simulink model "Aufgabe2_nicht_linear"  (R2025b)
settings: Solver=ode5  StartTime=0.0  StopTime=50  FixedStep=0.05  RelTol=1e-3
settings Model: Creator=henri  LastModifiedBy=henri

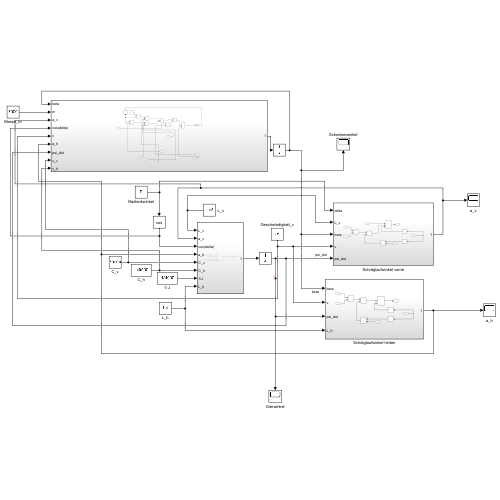
[thumbnail: Simulink's stored preview of the top-level diagram]
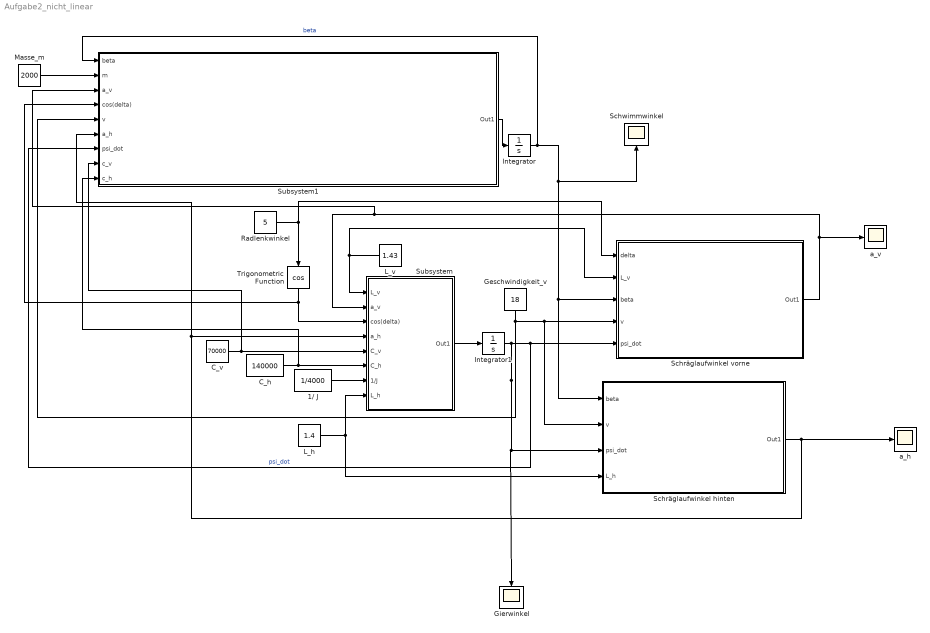
== system Aufgabe2_nicht_linear ==
  1/ J : Constant  Value=1/4000
  C_h : Constant  Value=140000
  C_v : Constant  Value=70000
  Geschwindigkeit_v : Constant  Value=18
  Gierwinkel : Scope
      settings: ActiveDisplayYMinimum=-1.0140786110140794  ActiveDisplayYMaximum=9.1267074991267165
  Integrator : Integrator
  Integrator1 : Integrator
  L_h : Constant  Value=1.4
  L_v : Constant  Value=1.43
  Masse_m : Constant  Value=2000
  Radlenkwinkel : Constant  Value=5
  Schräglaufwinkel hinten : Subsystem
  Schräglaufwinkel vorne : Subsystem
  Schwimmwinkel : Scope
      settings: ActiveDisplayYMinimum=-0.67350842338242578  ActiveDisplayYMaximum=0.35724955186258422
  Subsystem : Subsystem
  Subsystem1 : Subsystem
  Trigonometric Function : Trigonometry  Operator=cos
  a_h : Scope
      settings: ActiveDisplayYMinimum=0.59875782230441044  ActiveDisplayYMaximum=0.7625039748548651  DataLoggingVariableName=ScopeData2
  a_v : Scope
      settings: ActiveDisplayYMinimum=4.248464796495246  ActiveDisplayYMaximum=4.4144687229732016  DataLoggingVariableName=ScopeData3
  wires:
  Trigonometric Function/1 -> Subsystem1/4(cos(delta)), Subsystem/3(cos(delta))
  Radlenkwinkel/1 -> Trigonometric Function/1, Schräglaufwinkel vorne/1(delta)
  L_h/1 -> Subsystem/8(L_h), Schräglaufwinkel hinten/4(L_h)
  Integrator1/1 -> Gierwinkel/1, Schräglaufwinkel hinten/3(psi_dot), Subsystem1/7(psi_dot), Schräglaufwinkel vorne/5(psi_dot)  "psi_dot"
  L_v/1 -> Schräglaufwinkel vorne/2(L_v), Subsystem/1(L_v)
  C_v/1 -> Subsystem1/8(c_v), Subsystem/5(C_v)
  1/ J/1 -> Subsystem/7(1/J)
  Geschwindigkeit_v/1 -> Subsystem1/5(v), Schräglaufwinkel vorne/4(v), Schräglaufwinkel hinten/2(v)
  C_h/1 -> Subsystem1/9(c_h), Subsystem/6(C_h)
  Schräglaufwinkel vorne/1(Out1) -> a_v/1, Subsystem1/3(a_v), Subsystem/2(a_v)
  Subsystem/1(Out1) -> Integrator1/1
  Integrator/1 -> Subsystem1/1(beta), Schwimmwinkel/1, Schräglaufwinkel vorne/3(beta), Schräglaufwinkel hinten/1(beta)  "beta"
  Schräglaufwinkel hinten/1(Out1) -> Subsystem1/6(a_h), Subsystem/4(a_h), a_h/1
  Masse_m/1 -> Subsystem1/2(m)
  Subsystem1/1(Out1) -> Integrator/1

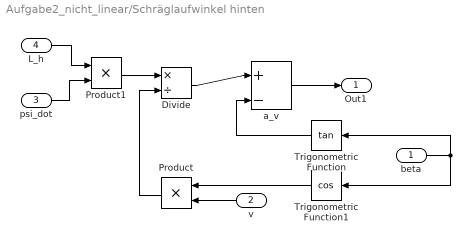
== system Aufgabe2_nicht_linear/Schräglaufwinkel hinten ==
  beta : Inport
  v : Inport  Port=2
  psi_dot : Inport  Port=3
  L_h : Inport  Port=4
  Divide : Product  Inputs=*/
  Product : Product
  Product1 : Product
  Trigonometric Function : Trigonometry  Operator=tan
  Trigonometric Function1 : Trigonometry  Operator=cos
  a_v : Sum  Inputs=|+-
  Out1 : Outport
  wires:
  L_h/1 -> Product1/1
  v/1 -> Product/2
  beta/1 -> Trigonometric Function1/1, Trigonometric Function/1
  psi_dot/1 -> Product1/2
  Trigonometric Function1/1 -> Product/1
  Product/1 -> Divide/2
  Product1/1 -> Divide/1
  Divide/1 -> a_v/1
  a_v/1 -> Out1/1
  Trigonometric Function/1 -> a_v/2

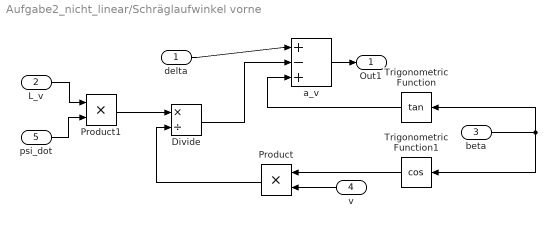
== system Aufgabe2_nicht_linear/Schräglaufwinkel vorne ==
  delta : Inport
  L_v : Inport  Port=2
  beta : Inport  Port=3
  v : Inport  Port=4
  psi_dot : Inport  Port=5
  Divide : Product  Inputs=*/
  Product : Product
  Product1 : Product
  Trigonometric Function : Trigonometry  Operator=tan
  Trigonometric Function1 : Trigonometry  Operator=cos
  a_v : Sum  Inputs=|+-+
  Out1 : Outport
  wires:
  Product/1 -> Divide/2
  Divide/1 -> a_v/2
  Trigonometric Function1/1 -> Product/1
  L_v/1 -> Product1/1
  v/1 -> Product/2
  Product1/1 -> Divide/1
  Trigonometric Function/1 -> a_v/3
  beta/1 -> Trigonometric Function1/1, Trigonometric Function/1
  delta/1 -> a_v/1
  a_v/1 -> Out1/1
  psi_dot/1 -> Product1/2

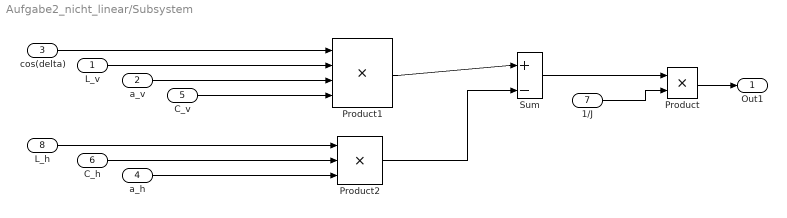
== system Aufgabe2_nicht_linear/Subsystem ==
  L_v : Inport
  a_v : Inport  Port=2
  cos(delta) : Inport  Port=3
  a_h : Inport  Port=4
  C_v : Inport  Port=5
  C_h : Inport  Port=6
  1/J : Inport  Port=7
  L_h : Inport  Port=8
  Product : Product
  Product1 : Product  Inputs=4
  Product2 : Product  Inputs=3
  Sum : Sum  Inputs=|+-
  Out1 : Outport
  wires:
  Product1/1 -> Sum/1
  Product2/1 -> Sum/2
  a_v/1 -> Product1/3
  1/J/1 -> Product/2
  Sum/1 -> Product/1
  cos(delta)/1 -> Product1/1
  Product/1 -> Out1/1
  a_h/1 -> Product2/3
  C_h/1 -> Product2/2
  L_h/1 -> Product2/1
  L_v/1 -> Product1/2
  C_v/1 -> Product1/4

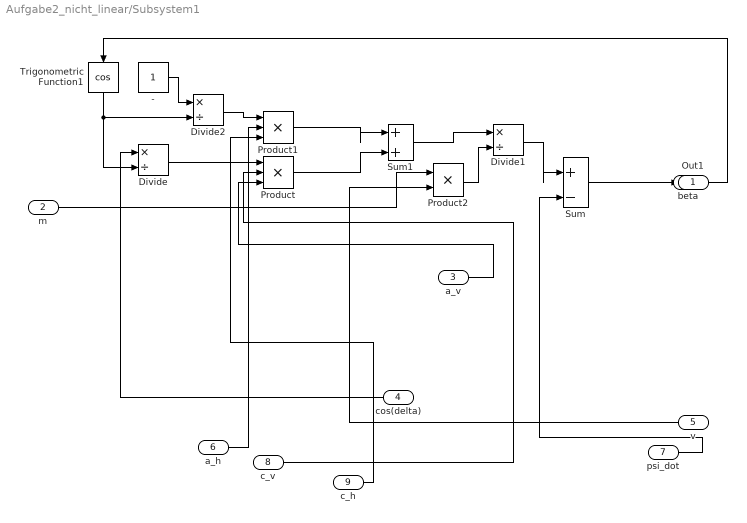
== system Aufgabe2_nicht_linear/Subsystem1 ==
  beta : Inport
  m : Inport  Port=2
  a_v : Inport  Port=3
  cos(delta) : Inport  Port=4
  v : Inport  Port=5
  a_h : Inport  Port=6
  psi_dot : Inport  Port=7
  c_v : Inport  Port=8
  c_h : Inport  Port=9
  - : Constant
  Divide : Product  Inputs=*/
  Divide1 : Product  Inputs=*/
  Divide2 : Product  Inputs=*/
  Product : Product  Inputs=3
  Product1 : Product  Inputs=3
  Product2 : Product
  Sum : Sum  Inputs=|+-
  Sum1 : Sum  Inputs=|++
  Trigonometric Function1 : Trigonometry  Operator=cos
  Out1 : Outport
  wires:
  Sum1/1 -> Divide1/1
  Product2/1 -> Divide1/2
  psi_dot/1 -> Sum/2
  Product/1 -> Sum1/2
  Product1/1 -> Sum1/1
  Divide/1 -> Product/1
  Divide2/1 -> Product1/1
  Trigonometric Function1/1 -> Divide2/2, Divide/2
  Divide1/1 -> Sum/1
  -/1 -> Divide2/1
  a_h/1 -> Product1/2
  c_h/1 -> Product1/3
  m/1 -> Product2/1
  cos(delta)/1 -> Divide/1
  a_v/1 -> Product/3
  c_v/1 -> Product/2
  Sum/1 -> Out1/1
  v/1 -> Product2/2
  beta/1 -> Trigonometric Function1/1
